simulink model "simulink1_dynamic"  (R2022a)
settings: Solver=FixedStepDiscrete  StartTime=0.0  StopTime=10.0  FixedStep=0.1  RelTol=1e-3
model workspace (MAT data in the model file):
  acceleration = 1
  alignment = 1
  cohesion = 1
  d_min = 0.5
  dt = 1
  eta = 1.5
  forward = 1
  k_ = 0.5
  k_tsmc = 1
  lambda_ = 2
  leader_position = [0 0 5]
  leader_velocity = [1 1 0]
  max_velocity = 5
  n_drones = 10
  neighbor_rad = 15
  radius = 10
  radius1 = 20
  ref_position = [20 20 5]
  ref_velocity = [0 0 0]
  separation = 1.5
  time_steps = 50
  u_max = 10
  velocities = [5 5 5]
  velocity = 5
settings Model: Creator=admin  LastModifiedBy=admin

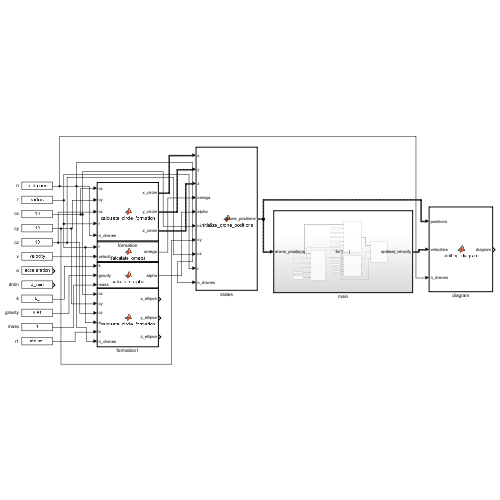
[thumbnail: Simulink's stored preview of the top-level diagram]
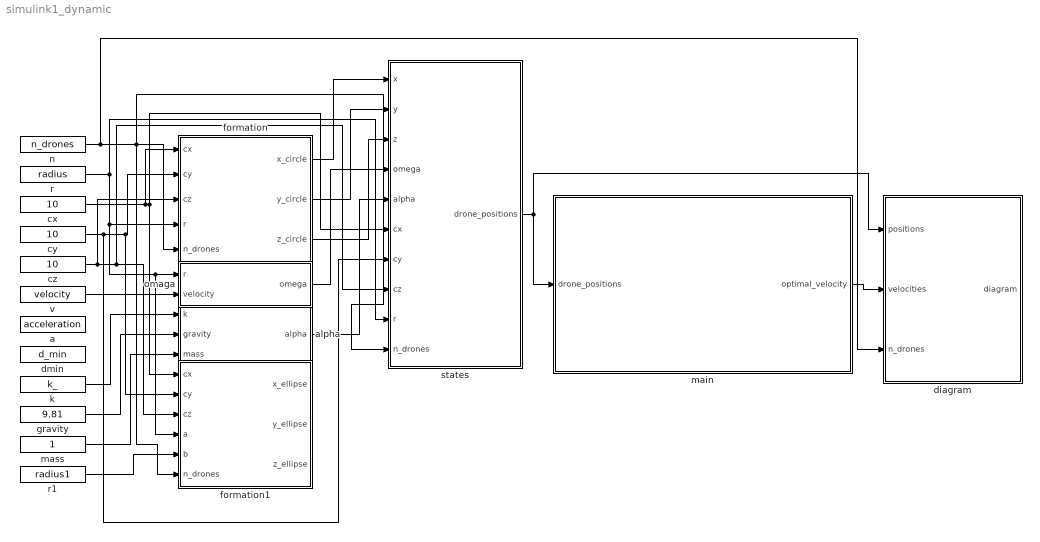
== system simulink1_dynamic ==
  a : Constant  Value=acceleration
  alpha : MATLAB Function  TreatAsAtomicUnit=on
  cx : Constant  Value=10
  cy : Constant  Value=10
  cz : Constant  Value=10
  diagram : MATLAB Function  TreatAsAtomicUnit=on
  dmin : Constant  Value=d_min
  formation : MATLAB Function  TreatAsAtomicUnit=on  SystemSampleTime=0.1
  formation1 : MATLAB Function  TreatAsAtomicUnit=on  SystemSampleTime=0.1
  gravity : Constant  Value=9.81
  k : Constant  Value=k_
  main : Subsystem  TreatAsAtomicUnit=on
  mass : Constant
  n : Constant  Value=n_drones
  omaga : MATLAB Function  TreatAsAtomicUnit=on
  r : Constant  Value=radius
  r1 : Constant  Value=radius1
  states : MATLAB Function  TreatAsAtomicUnit=on  SystemSampleTime=0.1
  v : Constant  Value=velocity
  wires:
  v/1 -> omaga/2(velocity)
  r/1 -> formation1/4(a), omaga/1(r), formation/4(r), states/9(r)
  k/1 -> alpha/1(k)
  gravity/1 -> alpha/2(gravity)
  mass/1 -> alpha/3(mass)
  cx/1 -> states/6(cx), formation1/1(cx), formation/1(cx)
  cy/1 -> states/7(cy), formation1/2(cy), formation/2(cy)
  cz/1 -> states/8(cz), formation1/3(cz), formation/3(cz)
  n/1 -> diagram/3(n_drones), states/10(n_drones), formation1/6(n_drones), formation/5(n_drones)
  r1/1 -> formation1/5(b)
  states/1(drone_positions) -> diagram/1(positions), main/1(drone_positions)
  formation/1(x_circle) -> states/1(x)
  formation/2(y_circle) -> states/2(y)
  formation/3(z_circle) -> states/3(z)
  omaga/1(omega) -> states/4(omega)
  alpha/1(alpha) -> states/5(alpha)
  main/1(optimal_velocity) -> diagram/2(velocities)

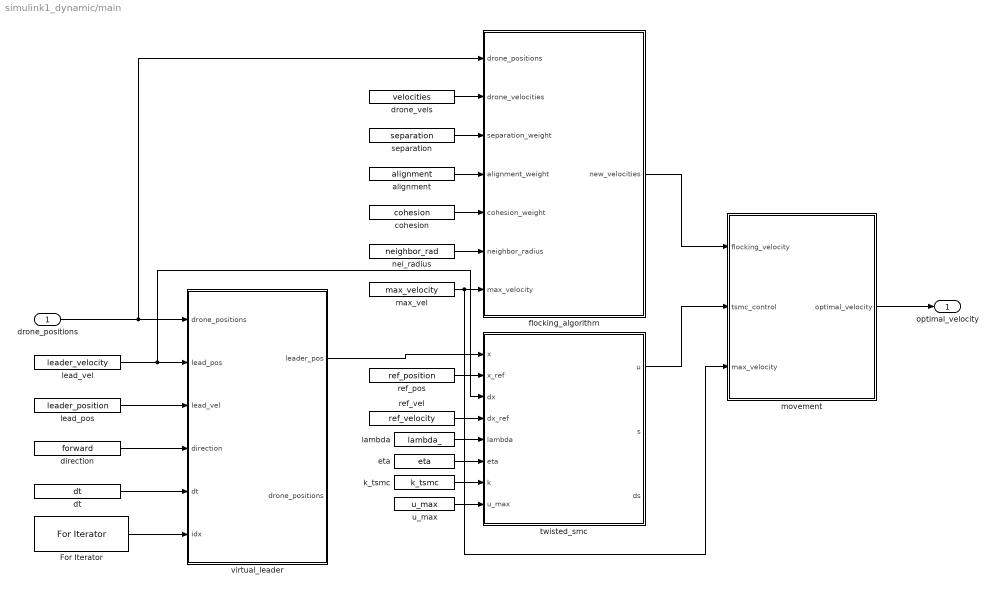
== system simulink1_dynamic/main ==
  drone_positions : Inport
  For Iterator : ForIterator  IterationLimit=time_steps
  alignment : Constant  Value=alignment
  cohesion : Constant  Value=cohesion
  direction : Constant  Value=forward
  drone_vels : Constant  Value=velocities
  dt : Constant  Value=dt
  eta : Constant  Value=eta
  flocking_algorithm : MATLAB Function  TreatAsAtomicUnit=on
  k_tsmc : Constant  Value=k_tsmc
  lambda : Constant  Value=lambda_
  lead_pos : Constant  Value=leader_position
  lead_vel : Constant  Value=leader_velocity
  max_vel : Constant  Value=max_velocity
  movement : MATLAB Function  TreatAsAtomicUnit=on
  nei_radius : Constant  Value=neighbor_rad
  ref_pos : Constant  Value=ref_position
  ref_vel : Constant  Value=ref_velocity
  separation : Constant  Value=separation
  twisted_smc : MATLAB Function  TreatAsAtomicUnit=on
  u_max : Constant  Value=u_max
  virtual_leader : MATLAB Function  TreatAsAtomicUnit=on
  optimal_velocity : Outport
  wires:
  dt/1 -> virtual_leader/5(dt)
  lead_vel/1 -> twisted_smc/3(dx), virtual_leader/2(lead_pos)
  direction/1 -> virtual_leader/4(direction)
  lead_pos/1 -> virtual_leader/3(lead_vel)
  drone_positions/1 -> flocking_algorithm/1(drone_positions), virtual_leader/1("drone_positions ")
  For Iterator/1 -> virtual_leader/6(idx)
  ref_vel/1 -> twisted_smc/4(dx_ref)
  ref_pos/1 -> twisted_smc/2(x_ref)
  virtual_leader/1(leader_pos) -> twisted_smc/1(x)
  lambda/1 -> twisted_smc/5(lambda)
  eta/1 -> twisted_smc/6(eta)
  k_tsmc/1 -> twisted_smc/7(k)
  u_max/1 -> twisted_smc/8(u_max)
  separation/1 -> flocking_algorithm/3(separation_weight)
  alignment/1 -> flocking_algorithm/4(alignment_weight)
  cohesion/1 -> flocking_algorithm/5(cohesion_weight)
  nei_radius/1 -> flocking_algorithm/6(neighbor_radius)
  max_vel/1 -> movement/3(max_velocity), flocking_algorithm/7(max_velocity)
  twisted_smc/1(u) -> movement/2(tsmc_control)
  flocking_algorithm/1(new_velocities) -> movement/1(flocking_velocity)
  drone_vels/1 -> flocking_algorithm/2(drone_velocities)
  movement/1(optimal_velocity) -> optimal_velocity/1

== matlab function simulink1_dynamic/main/virtual_leader ==
  data: drone_positions input; lead_pos input; leader_pos output; lead_vel input; direction input; dt input; drone_positions output; idx input
function [leader_pos, drone_positions] = virtual_leader(drone_positions, lead_pos, lead_vel, direction, dt, idx)
    switch direction
        case 1 % Forward
            lead_pos(1) = lead_pos(1) + lead_vel(1) * dt;
        case 2 % Backward
            lead_pos(1) = lead_pos(1) - lead_vel(1) * dt;
        case 3 % Left
            lead_pos(2) = lead_pos(2) - lead_vel(2) * dt;
        case 4 % Right
            lead_pos(2) = lead_pos(2) + lead_vel(2) * dt;
        case 5 % Up
            lead_pos(3) = lead_pos(3) + lead_vel(3) * dt;
        case 6 % Down
            lead_pos(3) = lead_pos(3) - lead_vel(3) * dt;
        otherwise
    end
    
    leader_pos = lead_pos;
end

== matlab function simulink1_dynamic/main/twisted_smc ==
  data: x input; u output; x_ref input; dx input; dx_ref input; lambda input; eta input; k input; u_max input; s output; ds output
function [u, s, ds] = twisted_sliding_control(x, x_ref, dx, dx_ref, lambda, eta, k, u_max)
    s = (x - x_ref) + lambda * (dx - dx_ref);
    ds = (dx - dx_ref) + lambda * (x - x_ref);

    u_eq = -lambda * dx;
    u_tsmc = k * sign(ds) - eta * sign(s);
    u = u_eq + u_tsmc;
    u = min(max(u, -u_max), u_max);
end

== matlab function simulink1_dynamic/main/flocking_algorithm ==
  data: drone_positions input; new_velocities output size=[1, 3]; drone_velocities input size=[1, 3]; separation_weight input; alignment_weight input; cohesion_weight input; neighbor_radius input; max_velocity input
function new_velocities = flocking_control_alpha_lattice(drone_positions, drone_velocities, separation_weight, alignment_weight, cohesion_weight, neighbor_radius, max_velocity)
    n_drones = size(drone_positions, 1);
    new_velocities = zeros(1, 3);
    
    for i = 1:n_drones
        current_position = drone_positions(i, :);

        separation_force = [0, 0, 0];
        alignment_force = [0, 0, 0];
        cohesion_force = [0, 0, 0];
        num_neighbors = 0;
        for j = 1:n_drones
            if i ~= j
                distance = norm(drone_positions(j, :) - current_position);
                if distance < neighbor_radius
                    separation_force = separation_force + (current_position - drone_positions(j, :)) / (distance^2);
                    alignment_force = alignment_force;
                    cohesion_force = cohesion_force + drone_positions(j, :);
                    num_neighbors = num_neighbors + 1;
                end
            end
        end

        if num_neighbors > 0
            alignment_force = (alignment_force / num_neighbors);
            alignment_force = alignment_weight * alignment_force;

            cohesion_force = (cohesion_force / num_neighbors) - current_position;
            cohesion_force = cohesion_weight * cohesion_force;

            separation_force = separation_weight * separation_force;
        end

        new_velocity = separation_force + alignment_force + cohesion_force;

        speed = norm(new_velocity);
        if speed > max_velocity
            new_velocity = (new_velocity / speed) * max_velocity;
        end

        new_velocities(1, :) = new_velocity;
    end
end

== matlab function simulink1_dynamic/main/movement ==
  data: flocking_velocity input size=[1, 3]; optimal_velocity output size=[n_drones, 3]; tsmc_control input; max_velocity input
function optimal_velocity = drone_movement(flocking_velocity, tsmc_control, max_velocity)
    tsmc_control = tsmc_control * ones(size(flocking_velocity));
    
    optimal_velocity = flocking_velocity + tsmc_control;

    speed = norm(optimal_velocity);
    if speed > max_velocity
        optimal_velocity = (optimal_velocity / speed) * max_velocity;
    end
end

== matlab function simulink1_dynamic/diagram ==
  data: positions input; velocities input; n_drones input; diagram output
function diagram = plotting_diagram(positions, velocities, n_drones)
    figure_handle = figure;
    r = 10;
    cx = 0;
    cy = 0;
    cz = 5;
    
    velocity = 5;
    dt = 1;
    total_time = 50;
    time_steps = total_time / dt;
    
    lambda = 2;
    eta = 1.5;
    k_tsmc = 1.0;
    u_max = 10;
    leader_velocity = [1, 1, 0];
    leader_position = [0, 0, 5];
    leader_ref_velocity = [0, 0, 0];
    leader_ref_position = [20, 20, 5];
    
    % Initialize drone positions and velocities
    x_circle = cx + r * cos((2 * pi * (0:n_drones-1)) / n_drones);
    y_circle = cy + r * sin((2 * pi * (0:n_drones-1)) / n_drones);
    z_circle = cz * ones(1, n_drones);
    drone_positions = [x_circle', y_circle', z_circle'];
    drone_velocities = zeros(n_drones, 3);
    
    % Flocking parameters
    separation_weight = 1.5;
    alignment_weight = 1.0;
    cohesion_weight = 1.0;
    neighbor_radius = 15;
    max_velocity = 5;
    
    % Simulation loop
    for t = 1:time_steps
        % Update leader's position and velocity using TSMC
        [u_x, u_y, u_z] = twisted_sliding_control(leader_position, leader_velocity, leader_ref_position, leader_ref_velocity, lambda, eta, k_tsmc, u_max);
        leader_velocity = [u_x, u_y, u_z];
        leader_position = leader_position + leader_velocity * dt;

        % Update each drone's flocking behavior
        for i = 1:n_drones
            [sep_force, align_force, cohes_force] = calculate_flocking_forces(drone_positions, drone_velocities, i, separation_weight, alignment_weight, cohesion_weight, neighbor_radius);
            drone_velocities(i, :) = apply_flocking(drone_velocities(i, :), sep_force, align_force, cohes_force, max_velocity);
        end

        % Update positions based on new velocities
        drone_positions = drone_positions + drone_velocities * dt;

        % Plot formation
        plot_formation(drone_positions, r, cx, cy, cz, t, dt, figure_handle);

        pause(0.1);
    end
    diagram = 1;  % Dummy output for Simulink decoration
end

% Twisted Sliding Mode Control (TSMC) helper functions
function [u_x, u_y, u_z] = twisted_sliding_control(position, velocity, ref_position, ref_velocity, lambda, eta, k, u_max)
    u_x = control_single_axis(position(1), velocity(1), ref_position(1), ref_velocity(1), lambda, eta, k, u_max);
    u_y = control_single_axis(position(2), velocity(2), ref_position(2), ref_velocity(2), lambda, eta, k, u_max);
    u_z = control_single_axis(position(3), velocity(3), ref_position(3), ref_velocity(3), lambda, eta, k, u_max);
end

function u = control_single_axis(x, dx, x_ref, dx_ref, lambda, eta, k, u_max)
    s = (x - x_ref) + lambda * (dx - dx_ref);
    ds = (dx - dx_ref) + lambda * (x - x_ref);
    u_eq = -lambda * dx;
    u_tsmc = k * sign(ds) - eta * sign(s);
    u = u_eq + u_tsmc;
    u = min(max(u, -u_max), u_max);
end

% Flocking behavior helper functions
function [sep_force, align_force, cohes_force] = calculate_flocking_forces(drone_positions, drone_velocities, drone_index, separation_weight, alignment_weight, cohesion_weight, neighbor_radius)
    current_position = drone_positions(drone_index, :);
    current_velocity = drone_velocities(drone_index, :);
    sep_force = [0, 0, 0];
    align_force = [0, 0, 0];
    cohes_force = [0, 0, 0];
    num_neighbors = 0;

    for i = 1:size(drone_positions, 1)
        if i ~= drone_index
            distance = norm(drone_positions(i, :) - current_position);
            if distance < neighbor_radius
                sep_force = sep_force + (current_position - drone_positions(i, :)) / (distance^2);
                align_force = align_force + drone_velocities(i, :);
                cohes_force = cohes_force + drone_positions(i, :);
                num_neighbors = num_neighbors + 1;
            end
        end
    end

    if num_neighbors > 0
        align_force = alignment_weight * ((align_force / num_neighbors) - current_velocity);
        cohes_force = cohesion_weight * ((cohes_force / num_neighbors) - current_position);
        sep_force = separation_weight * sep_force;
    end
end

function new_velocity = apply_flocking(current_velocity, sep_force, align_force, cohes_force, max_velocity)
    new_velocity = current_velocity + sep_force + align_force + cohes_force;
    speed = norm(new_velocity);
    if speed > max_velocity
        new_velocity = (new_velocity / speed) * max_velocity;
    end
end

function plot_formation(drone_positions, r, cx, cy, cz, t, dt, figure_handle)
    persistent previous_formation active_drones;
    
    if isempty(previous_formation)
        n_drones = 10;
        previous_formation = [cx + rand(1, n_drones)' * r, cy + rand(1, n_drones)' * r, cz * ones(n_drones, 1)];
        active_drones = n_drones;
    end

    if t <= 20
        active_drones = 10;
    elseif t > 20 && t <= 30
        active_drones = max(4, active_drones - 1);
    elseif t > 30 && t <= 40
        active_drones = min(10, active_drones + 1);
    end

    n_drones = size(previous_formation, 1);
    centroid = mean(previous_formation, 1);
    
    if t <= 16
        x_target = linspace(centroid(1) - r, centroid(1) + r, n_drones);
        y_target = centroid(2) * ones(1, n_drones);
        z_target = centroid(3) * ones(1, n_drones);
        outer_shape = 'line';
    elseif t <= 33
        x_target = centroid(1) + r * cos((2 * pi * (0:n_drones-1)) / n_drones);
        y_target = centroid(2) + r * sin((2 * pi * (0:n_drones-1)) / n_drones);
        z_target = centroid(3) * ones(1, n_drones);
        outer_shape = 'circle';
    elseif t <= 49
        x_target = centroid(1) + (r * 1.5) * cos((2 * pi * (0:n_drones-1)) / n_drones);
        y_target = centroid(2) + r * sin((2 * pi * (0:n_drones-1)) / n_drones);
        z_target = centroid(3) * ones(1, n_drones);
        outer_shape = 'ellipse';
    else
        x_target = centroid(1) + (r * 1.5) * cos((2 * pi * (0:n_drones-1)) / n_drones);
        y_target = centroid(2) + r * sin((2 * pi * (0:n_drones-1)) / n_drones);
        z_target = centroid(3) * ones(1, n_drones);
        outer_shape = 'ellipse';
    end

    for i = 1:n_drones
        if i > active_drones
            x_target(i) = x_target(i) + 10 * sign(x_target(i) - centroid(1));
            y_target(i) = y_target(i) + 10 * sign(y_target(i) - centroid(2));
        end
    end

    smoothing_factor = 0.5;
    x_formation = previous_formation(:, 1)' + (x_target - previous_formation(:, 1)') * smoothing_factor;
    y_formation = previous_formation(:, 2)' + (y_target - previous_formation(:, 2)') * smoothing_factor;
    z_formation = previous_formation(:, 3)' + (z_target - previous_formation(:, 3)') * smoothing_factor;

    previous_formation = [x_formation', y_formation', z_formation'];

    figure(figure_handle);
    clf;

    plot3(x_formation(1:active_drones), y_formation(1:active_drones), z_formation(1:active_drones), 'ro', 'MarkerSize', 5);
    hold on;
    
    for i = 1:active_drones
        next_index = mod(i, active_drones) + 1;
        plot3([x_formation(i), x_formation(next_index)], ...
              [y_formation(i), y_formation(next_index)], ...
              [z_formation(i), z_formation(next_index)], ...
              'r-');
    end
   
    theta = linspace(0, 2 * pi, 100);
    x_outer = zeros(1, 100);
    y_outer = zeros(1, 100);
    z_outer = zeros(1, 100);

    switch outer_shape
        case 'line'
            x_outer = linspace(centroid(1) - r, centroid(1) + r, 100);
            y_outer = centroid(2) * ones(1, 100);
            z_outer = centroid(3) * ones(1, 100);
        case 'circle'
            x_outer = centroid(1) + r * cos(theta);
            y_outer = centroid(2) + r * sin(theta);
            z_outer = centroid(3) * ones(1, length(theta));
        case 'ellipse'
            x_outer = centroid(1) + (r * 1.5) * cos(theta);
            y_outer = centroid(2) + r * sin(theta);
            z_outer = centroid(3) * ones(1, length(theta));
    end
    
    plot3(x_outer, y_outer, z_outer, 'k--', 'LineWidth', 1);

    if t <= 16
        text(x_formation(1), y_formation(1), z_formation(1), 'Line Formation', 'Color', 'red');
    elseif t <= 33
        text(x_formation(1), y_formation(1), z_formation(1), 'Circle Formation', 'Color', 'red');
    elseif t <= 49
        text(x_formation(1), y_formation(1), z_formation(1), 'Ellipsis Formation', 'Color', 'red');
    else
        text(x_formation(1), y_formation(1), z_formation(1), 'Spiral Formation', 'Color', 'red');
    end
    
    xlabel('X');
    ylabel('Y');
    zlabel('Z');
    title(['Time: ', sprintf('%0.2f', t * dt)]);
    axis equal;
    grid on;
    axis([-40 40 -40 40 0 40]);
    drawnow;
end

== matlab function simulink1_dynamic/alpha ==
  data: k input; alpha output; gravity input; mass input
function alpha = calculate_alpha(k, gravity, mass)
    alpha = k * (gravity / mass);
end

== matlab function simulink1_dynamic/omaga ==
  data: r input; velocity input; omega output
function omega = calculate_omega(r, velocity)
    omega = (2 * pi * velocity) / r;
end

== matlab function simulink1_dynamic/formation ==
  data: cx input; x_circle output size=[1, n_drones]; cy input; cz input; r input; n_drones input; y_circle output size=[1, n_drones]; z_circle output size=[1, n_drones]
function [x_circle, y_circle, z_circle] = calculate_circle_formation(cx, cy, cz, r, n_drones)
    theta = (2 * pi * (0:n_drones-1)) / n_drones;
    
    x_circle = cx + r * cos(theta);
    y_circle = cy + r * sin(theta);
    z_circle = cz * ones(1, n_drones);
end

== matlab function simulink1_dynamic/formation1 ==
  data: cx input; x_ellipse output size=[1, n_drones]; cy input; cz input; a input; b input; n_drones input; y_ellipse output size=[1, n_drones]; z_ellipse output size=[1, n_drones]
function [x_ellipse, y_ellipse, z_ellipse] = calculate_circle_formation(cx, cy, cz, a, b, n_drones)
    
    x_ellipse = cx + a * cos((2 * pi * (0:n_drones-1)) / n_drones);
    y_ellipse = cy + b * sin((2 * pi * (0:n_drones-1)) / n_drones);
    z_ellipse = cz * ones(1, n_drones);

end

== matlab function simulink1_dynamic/states ==
  data: x input; y input; z input; omega input; alpha input; cx input; drone_positions output size=[n_drones, 3]; cy input; cz input; r input; n_drones input
function drone_positions = initialize_drone_positions(x, y, z, omega, alpha, cx, cy, cz, r, n_drones)
    theta = (2 * pi * (0:n_drones-1)) / n_drones;
    
    x_positions = cx + r * cos(theta); % 1 x n_drones
    y_positions = cy + r * sin(theta); % 1 x n_drones
    z_positions = cz * ones(1, n_drones); % 1 x n_drones
    
    drone_positions = [x_positions; y_positions; z_positions]';
end
